simulink model "solar_panal"  (R2022b)
settings: Solver=VariableStepAuto  StartTime=0.0  StopTime=15*3600  RelTol=1e-3
model workspace (MAT data in the model file):
  kd = 5
  l = 5
libraries: slpidlib x1
settings Model: Creator=yasso  LastModifiedBy=yasso
settings DataIOCC: ExternalInput=[sunTime, sunPosition]  LoadExternalInput=on

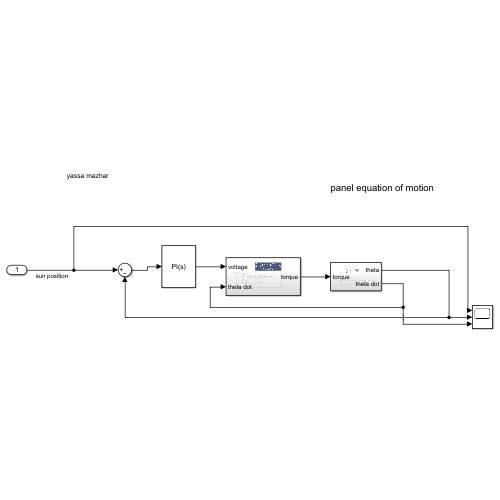
[thumbnail: Simulink's stored preview of the top-level diagram]
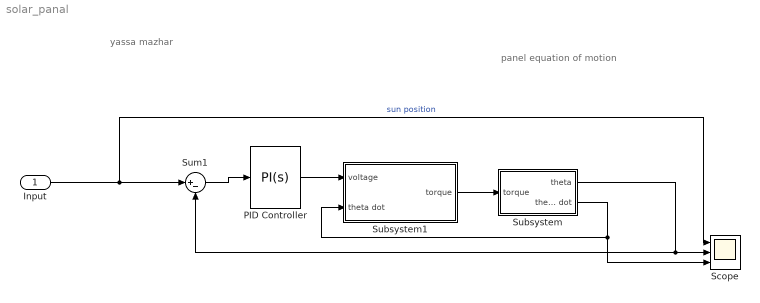
== system solar_panal ==
  note: yassa mazhar
  note: panel equation of motion
  Input : Inport
  PID Controller : slpidlib/PID Controller  Controller=PI  Form=Parallel  TimeDomain=Continuous-time  UseExternalTs=off  SampleTime=-1  IntegratorMethod=Forward Euler  FilterMethod=Forward Euler  ControllerParametersSource=internal  P=240  I=180  UseKiTs=off  D=0  N=100  UseFilter=on  TunerSelectOption=Transfer Function Based (PID Tuner App)  InitialConditionSource=internal  InitialConditionForIntegrator=0  InitialConditionForFilter=0  DifferentiatorICPrevScaledInput=0  ExternalReset=none  TrackingMode=off  Kt=1  LimitOutput=off  SatLimitsSource=internal  UpperSaturationLimit=inf  LowerSaturationLimit=-inf  LinearizeAsGain=on  AntiWindupMode=none  Kb=1  LimitIntegrator=off  UpperIntegratorSaturationLimit=inf  LowerIntegratorSaturationLimit=-inf  POutMin=[]  POutMax=[]  IOutMin=[]  IOutMax=[]  DOutMin=[]  DOutMax=[]  NOutMin=[]  NOutMax=[]  SumOutMin=[]  SumOutMax=[]  SaturationOutMin=[]  SaturationOutMax=[]  PParamMin=[]  PParamMax=[]  IParamMin=[]  IParamMax=[]  DParamMin=[]  DParamMax=[]  NParamMin=[]  NParamMax=[]  KbParamMin=[]  KbParamMax=[]  KtParamMin=[]  KtParamMax=[]  KbOutMin=[]  KbOutMax=[]  KtOutMin=[]  KtOutMax=[]  IntegratorOutMin=[]  IntegratorOutMax=[]  FilterOutMin=[]  FilterOutMax=[]  SumI1OutMin=[]  SumI1OutMax=[]  SumI2OutMin=[]  SumI2OutMax=[]  SumI3OutMin=[]  SumI3OutMax=[]  SumI4OutMin=[]  SumI4OutMax=[]  SumDOutMin=[]  SumDOutMax=[]  DifferentiatorOutMin=[]  DifferentiatorOutMax=[]  FilterDiffOutCoefMin=[]  FilterDiffOutCoefMax=[]  ReciprocalOutMin=[]  ReciprocalOutMax=[]  SumDenOutMin=[]  SumDenOutMax=[]  SumNumOutMin=[]  SumNumOutMax=[]  DivideOutMin=[]  DivideOutMax=[]  UdiffTsProdOutMin=[]  UdiffTsProdOutMax=[]  NTsProdOutMin=[]  NTsProdOutMax=[]  UintegralTsProdOutMin=[]  UintegralTsProdOutMax=[]  UngainTsProdOutMin=[]  UngainTsProdOutMax=[]  ClampingZeroOutDataTypeStr=Inherit: Inherit via back propagation  ClampingZeroOutMin=[]  ClampingZeroOutMax=[]  FilterDenConstantOutDataTypeStr=Inherit: Inherit via back propagation  FilterDenConstantOutMin=[]  FilterDenConstantOutMax=[]  PCopyOutDataTypeStr=Inherit: Inherit via back propagation  PCopyOutMin=[]  PCopyOutMax=[]  NCopyOutDataTypeStr=Inherit: Inherit via back propagation  NCopyOutMin=[]  NCopyOutMax=[]  IntegratorContinuousStateAttributes=''  IntegratorStateMustResolveToSignalObject=off  IntegratorRTWStateStorageClass=Auto  FilterContinuousStateAttributes=''  FilterStateMustResolveToSignalObject=off  FilterRTWStateStorageClass=Auto  ParallelPVariant=InternalParameters  IdealPVariant=Disabled  IVariant=InternalParameters  DVariant=Disabled  IntegratorVariant=Continuous  SatVariant=Disabled  AWVariant=Passthrough  PCopyVariant=Disabled  TRVariant=Disabled  FdbkBlocksVariant=Forward  IdealPFdbkVariant=Disabled  SatFdbkVariant=Disabled  DerivativeFilterVariant=Disabled  NVariant=Disabled  NCopyVariant=Disabled_SignalSpec  FilterICVariant=Disabled  IntegratorICVariant=InternalICs  ExternalResetVariant=Disabled  TRSumVariant=Passthrough  SumFdbkVariant=Disabled  SumVariant=Sum_PI  TsampFilterVariant=InternalTs  TsampNgainVariant=Passthrough  TsampIntegralVariant=Passthrough  ExternalSaturationOutDataTypeStr=Inherit: Same as second input
  Scope : Scope  NumInputPorts=3
  Subsystem : Subsystem
  Subsystem1 : Subsystem
  Sum1 : Sum  Inputs=|+-
  wires:
  Subsystem1/1(torque) -> Subsystem/1(torque)
  Subsystem/1(theta) -> Sum1/2, Scope/2
  Subsystem/2(theta dot) -> Scope/3, Subsystem1/2(theta dot)
  Input/1 -> Scope/1, Sum1/1  "sun position"
  Sum1/1 -> PID Controller/1
  PID Controller/1 -> Subsystem1/1(voltage)

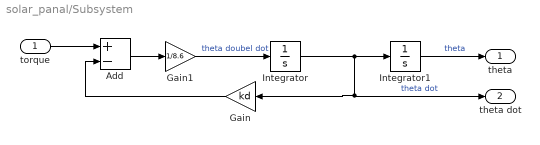
== system solar_panal/Subsystem ==
  torque : Inport
  Add : Sum  Inputs=+-
  Gain : Gain  Gain=kd
  Gain1 : Gain  Gain=1/8.6
  Integrator : Integrator
  Integrator1 : Integrator
  theta : Outport
  theta dot : Outport  Port=2
  wires:
  Integrator1/1 -> theta/1  "theta"
  Integrator/1 -> theta dot/1, Gain/1, Integrator1/1  "theta dot"
  Add/1 -> Gain1/1
  Gain/1 -> Add/2
  torque/1 -> Add/1
  Gain1/1 -> Integrator/1  "theta doubel dot"

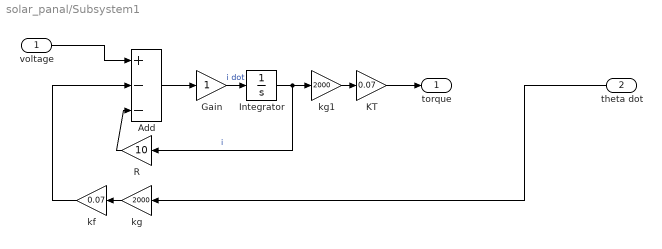
== system solar_panal/Subsystem1 ==
  voltage : Inport
  theta dot : Inport  Port=2
  Add : Sum  Inputs=+--
  Gain : Gain
  Integrator : Integrator
  KT : Gain  Gain=0.07
  R : Gain  Gain=10
  kf : Gain  Gain=0.07
  kg : Gain  Gain=2000
  kg1 : Gain  Gain=2000
  torque : Outport
  wires:
  kg1/1 -> KT/1
  kg/1 -> kf/1
  Add/1 -> Gain/1
  voltage/1 -> Add/1
  Gain/1 -> Integrator/1  "i dot"
  kf/1 -> Add/2
  R/1 -> Add/3
  Integrator/1 -> kg1/1, R/1  "i"
  KT/1 -> torque/1
  theta dot/1 -> kg/1
